simulink model "lqr_period_afbs_simu_thesis"  (R2015a)
settings: Solver=ode45  SolverMode=SingleTasking  StartTime=0.0  StopTime=simu.time  RelTol=1e-3
values from neighbouring files (symbols this model uses):
  A = importdata(filename,delimiterIn,headerlinesIn)    [analysis_pi_from_log.m]    (also in lqr_period_afbs.m = plant.model_ss.a; lqr_period_ideal_m.m = plant.model_ss.a; plot_pi_from_log.m)
  B = plant.model_ss.b    [lqr_period_afbs.m]    (also in lqr_period_ideal_m.m)
  C = plant.model_ss.c    [lqr_period_afbs.m]    (also in lqr_period_ideal_m.m)
undefined symbols (not defined in the file): afbs_parameters
settings Model: CovSFcnEnable=off  ExtModeTrigMode=oneshot  ExtModeArmWhenConnect=off  Creator=The MathWorks Inc.  LastModifiedBy=Steven
settings DataIOCC: LimitDataPoints=off  SaveOutput=off  SignalLogging=off  DSMLogging=off  SaveTime=off  SignalLoggingName=sigsOut
settings OptimizationCC: BooleanDataType=off  ExpressionDepthLimit=2147483647  InitFltsAndDblsToZero=on
settings DebuggingCC: SaveWithParameterizedLinksMsg=none  UnderspecifiedInitializationDetection=Classic  MergeDetectMultiDrivingBlocksExec=none  SignalResolutionControl=TryResolveAllWithWarning  MultiTaskDSMMsg=warning  MultiTaskCondExecSysMsg=none  IntegerOverflowMsg=none  FcnCallInpInsideContextMsg=UseLocalSettings  StateNameClashWarn=warning  IntegerSaturationMsg=none
settings HardwareCC: TargetUnknown=on
settings GRTTargetCC: TargetFcnLib=ansi_tfl_tmw.mat  CombineOutputUpdateFcns=off  GRTInterface=on

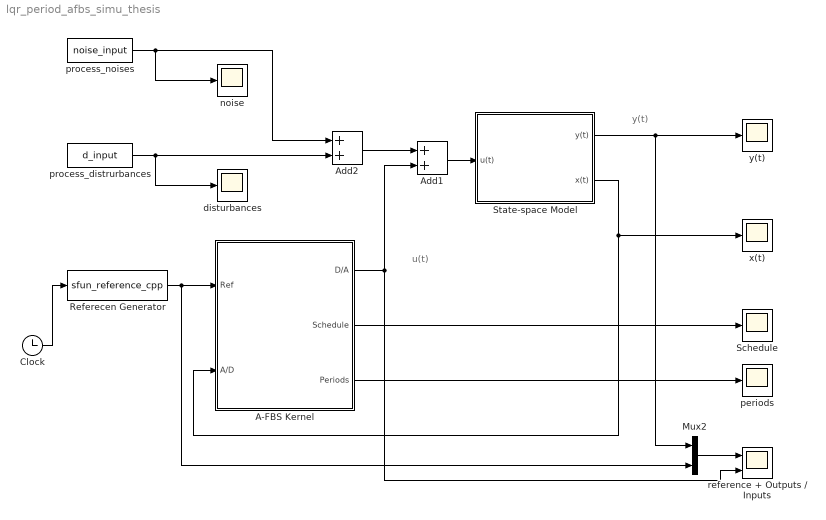
== system lqr_period_afbs_simu_thesis ==
  note: u(t)
  note: y(t)
  A-FBS Kernel : Subsystem  mask{para=afbs_parameters}
      mask prompts: para "A-FBS Parameters"
  Add1 : Sum
  Add2 : Sum
  Clock : Clock
  Mux2 : Mux  Inputs=2
  Referecen Generator : S-Function  FunctionName=sfun_reference_cpp
  Schedule : Scope
      settings: TimeRange=10  YMin=-29.95  YMax=-29.6  SaveName=ScopeData5  DataFormat=Structure  SampleTime=simu.samlping_time
  State-space Model : Subsystem  mask(State-space){A=A, B=B, C=C}
      mask help:
      | A state-space block using raw Simulink elements.
      | Internal states are exposed to use.
  disturbances : Scope
      settings: TimeRange=10  YMin=-29.95  YMax=-29.6  SaveName=ScopeData4  DataFormat=Structure  SampleTime=simu.sampling_time
  noise : Scope
      settings: TimeRange=10  YMin=-29.95  YMax=-29.6  SaveName=ScopeData3  DataFormat=Structure  SampleTime=simu.samlping_time
  periods : Scope
      settings: TimeRange=10  YMin=0.00095  YMax=0.00105  SaveName=ScopeData6  DataFormat=Structure  SampleTime=simu.samlping_time
  process_distrurbances : FromWorkspace  VariableName=d_input  SampleTime=0
  process_noises : FromWorkspace  VariableName=noise_input  SampleTime=0
  reference + Outputs / Inputs : Scope  NumInputPorts=2
      settings: TimeRange=1.022054868208716  YMin=-1~-0.1  YMax=7~0.7000000000000001  DataFormat=Structure  SampleTime=simu.samlping_time
  x(t) : Scope
      settings: TimeRange=10  YMin=0.00095  YMax=0.00105  SaveName=ScopeData2  DataFormat=Structure  SampleTime=simu.samlping_time
  y(t) : Scope
      settings: TimeRange=10  YMin=-1.5  YMax=1.75  DataFormat=Structure
  wires:
  A-FBS Kernel/1(D/A) -> reference + Outputs / Inputs/2, Add1/2
  State-space Model/1(y(t)) -> Mux2/1, y(t)/1
  process_noises/1 -> Add2/1, noise/1
  Add1/1 -> State-space Model/1(u(t))
  process_distrurbances/1 -> disturbances/1, Add2/2
  Mux2/1 -> reference + Outputs / Inputs/1
  A-FBS Kernel/3(Periods) -> periods/1
  A-FBS Kernel/2(Schedule) -> Schedule/1
  Referecen Generator/1 -> Mux2/2, A-FBS Kernel/1(Ref)
  Add2/1 -> Add1/1
  State-space Model/2(x(t)) -> x(t)/1, A-FBS Kernel/2(A/D)
  Clock/1 -> Referecen Generator/1

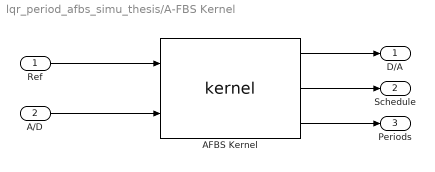
== system lqr_period_afbs_simu_thesis/A-FBS Kernel ==
  Ref : Inport
  A/D : Inport  Port=2
  AFBS Kernel : S-Function  FunctionName=kernel  Parameters=para
  D/A : Outport
  Schedule : Outport  Port=2
  Periods : Outport  Port=3
  wires:
  Ref/1 -> AFBS Kernel/1
  A/D/1 -> AFBS Kernel/2
  AFBS Kernel/2 -> Schedule/1
  AFBS Kernel/1 -> D/A/1
  AFBS Kernel/3 -> Periods/1

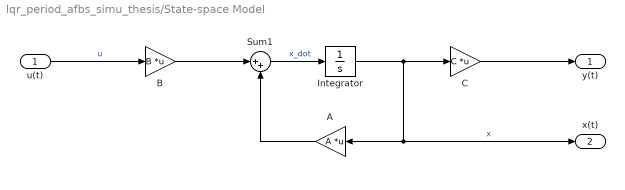
== system lqr_period_afbs_simu_thesis/State-space Model ==
  u(t) : Inport
  A : Gain  Gain=A  Multiplication=Matrix(K*u)
  B : Gain  Gain=B  Multiplication=Matrix(K*u)
  C : Gain  Gain=C  Multiplication=Matrix(K*u)
  Integrator : Integrator
  Sum1 : Sum  Inputs=|++
  y(t) : Outport
  x(t) : Outport  Port=2
  wires:
  u(t)/1 -> B/1  "u"
  B/1 -> Sum1/1
  A/1 -> Sum1/2
  Sum1/1 -> Integrator/1  "x_dot"
  Integrator/1 -> A/1, x(t)/1, C/1  "x"
  C/1 -> y(t)/1
